simulink model "BO_realisation"  (R2021a)
settings: Solver=FixedStepAuto  StartTime=0.0  StopTime=inf  FixedStep=0.1  RelTol=1e-3  EnableMultiTasking=on
InitFcn:
  | Ts=0.1;
undefined symbols (not defined in the file): sigbuilder_block
libraries: simulink x2, arduinolib x2
settings Model: SimulationMode=external  SILPILModeSetting=veronly  ExtModeTrigDuration=2  Creator=PHAN DU  LastModifiedBy=anass
settings SolverCC: AlgebraicLoopSolver=TrustRegion  AutoInsertRateTranBlk=on
settings DataIOCC: ReturnWorkspaceOutputs=off
settings OptimizationCC: EnhancedBackFolding=on  PassReuseOutputArgsAs=Individual arguments  ZeroExternalMemoryAtStartup=off  ZeroInternalMemoryAtStartup=off  MaxStackSize=64  OptimizeBlockOrder=speed  DifferentSizesBufferReuse=on  EfficientTunableParamExpr=on
settings DebuggingCC: ParameterTunabilityLossMsg=error  SFMachineParentedDataDiag=warning
settings HardwareCC: ProdBitPerInt=16  ProdBitPerPointer=16  ProdBitPerSizeT=16  ProdBitPerPtrDiffT=16  ProdLargestAtomicFloat=None  ProdWordSize=8  ProdHWDeviceType=Atmel->AVR
settings SFSimCC: MATLABDynamicMemAlloc=off
settings RTWCC: SystemTargetFile=ert.tlc  HardwareBoard=Arduino Mega 2560  TemplateMakefile=ert_default_tmf  Toolchain=Arduino AVR  BuildConfiguration=Faster Runs
settings CodeAppCC: ForceParamTrailComments=on  IgnoreCustomStorageClasses=off  OperatorAnnotations=on  SimulinkDataObjDesc=on  SFDataObjDesc=on  InsertBlockDesc=on
settings ERTTargetCC: SupportContinuousTime=on  SupportVariableSizeSignals=on  ExtMode=on  ExtModeStaticAllocSize=2048  ExtModeMexArgs='127.0.0.1' 0 17725

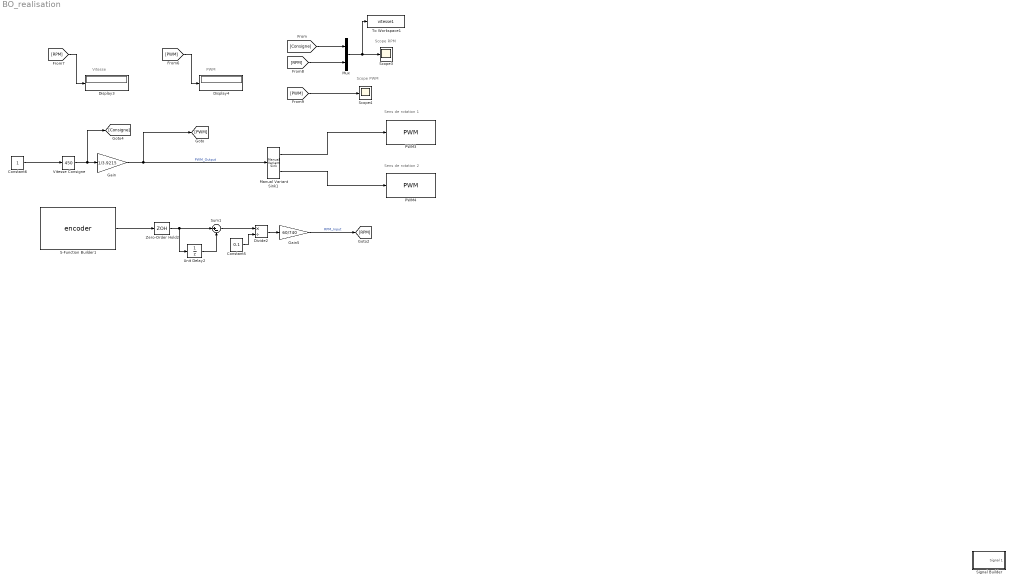
== system BO_realisation ==
  note: Scope PWM
  note: PWM
  note: Vitesse
  note: Scope RPM
  note: Sens de rotation 1
  note: Sens de rotation 2
  Constant5 : Constant  Value=0.1  SampleTime=0.1
  Constant6 : Constant
  Display3 : Display
  Display4 : Display
  Divide2 : Product  Inputs=*/
  Gain : Gain  Gain=1/3.9215
  Gain5 : Gain  Gain=60/740
  Manual Variant Sink1 : simulink/Signal Routing/Manual Variant Sink  NumChoices=2  LabelModeActiveChoice=V_2
  Mux : Mux  Inputs=2
  PWM3 : arduinolib/PWM  pinNumber=5  frequencyType=Default  desiredFrequency=490.2  achievableFrequency=2
  PWM4 : arduinolib/PWM  pinNumber=6  frequencyType=Default  desiredFrequency=490.2  achievableFrequency=2
  S-Function Builder1 : S-Function  InitFcn=try, set_param(gcb,'FunctionName','encoder'), end  FunctionName=encoder  Parameters=int8(0),int8(2),int8(3)  SFunctionModules=encoder_wrapper  SFunctionDeploymentMode=off  EnableBusSupport=off  mask(S-Function Builder){}
      mask help: Simulink:masks:SFunctionBuilder_MD
      mask init:
      | val = [[.9  0.75 0.75 1 1 .9 .9 1]',[1 1 0.75 0.75 .9 .9 1 .9]'];try , sys = get_param(gcb,'SfunBuilderFcnName');if isempty(sys), sys = get_param(gcb,'FunctionName'); end,catch, sys = get_param(gcb,'FunctionName'); end
      settings: CopyFcn=set_param(gcbh,'LinkStatus','none')  PreSaveFcn=try, set_param(gcb,'FunctionName','encoder'), end  OpenFcn=sfunctionwizard(gcbh)
      mask Display:
      | plot(val(:,1),val(:,2))
      | disp(sys)
      | port_label('output',1,'pos')
  Scope3 : Scope
  Scope4 : Scope
  Sum1 : Sum  Inputs=|+-
  To Workspace1 : ToWorkspace  VariableName=vitesse1  SaveFormat=Timeseries  SampleTime=-1
  Unit Delay2 : UnitDelay  SampleTime=-1  HasFrameUpgradeWarning=on
  "Vitesse Consigne " : simulink/Math Operations/Slider Gain  gain=450  low=0  high=1000
  Zero-Order Hold2 : ZeroOrderHold  SampleTime=0.1
  Signal Builder : Subsystem  Tag=STV Subsys  IOType=siggen  LoadFcn=sigbuilder_block('load');  StartFcn=sigbuilder_block('start');  StopFcn=sigbuilder_block('stop');  ClipboardFcn=sigbuilder_block('clipboard');  mask(Sigbuilder block){tuvar=[0:10]}
      mask help: Sigbuilder GUI
      mask init:
      | if ~strcmp(get_param(bdroot(gcbh),'SimulationStatus'),'stopped') tuvar = sigbuilder_block('maskInit'); end
      settings: CopyFcn=sigbuilder_block('copy');  DeleteFcn=sigbuilder_block('delete');  ModelCloseFcn=sigbuilder_block('modelClose');  PreSaveFcn=sigbuilder_block('preSave');  PauseFcn=sigbuilder_block('pause');  ContinueFcn=sigbuilder_block('continue');  NameChangeFcn=sigbuilder_block('namechange');  OpenFcn=sigbuilder_block('open',[437.6 199.2 550.4 400 ]);  CloseFcn=sigbuilder_block('close');
      mask Display: plot(0, 0, 100, 100,[2, 2, 32, 32, 2], [68, 8, 8, 68, 68],[32, 2], [38, 38], [32, 19, 2],[53, 60, 44], [32, 17, 17, 2],[16, 16, 31, 31]);txt = getActiveGroup(gcbh);text(2, 100, txt,'verticalAlignment', 'top');
  wires:
  Sum1/1 -> Divide2/1
  Gain5/1 -> [RPM]  "RPM_Input"
  Unit Delay2/1 -> Sum1/2
  Divide2/1 -> Gain5/1
  S-Function Builder1/1 -> Zero-Order Hold2/1
  [PWM] -> Display4/1
  Constant5/1 -> Divide2/2
  [PWM] -> Scope4/1
  Zero-Order Hold2/1 -> Sum1/1, Unit Delay2/1
  [RPM] -> Display3/1
  Constant6/1 -> "Vitesse Consigne "/1
  [Consigne] -> Mux/1
  [RPM] -> Mux/2
  "Vitesse Consigne "/1 -> [Consigne], Gain/1
  Manual Variant Sink1/2 -> PWM4/1
  Gain/1 -> Manual Variant Sink1/1, [PWM]  "PWM_Output"
  Manual Variant Sink1/1 -> PWM3/1
  Mux/1 -> To Workspace1/1, Scope3/1

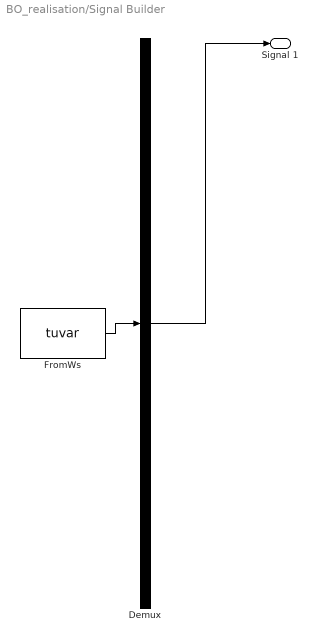
== system BO_realisation/Signal Builder ==
  Demux : Demux  Tag=STV Demux  Outputs=1
      settings: DisplayOption=none
  FromWs : FromWorkspace  Tag=STV FromWs  VariableName=tuvar
      SigBuilderData=|
      | common.afterFinalStr = 'Extrapolate'
      | common.sampleTime = 0
      | dataSet.timeRange = [0 10]
      | dataSet.name = 'Group 1'
      | sbobj.Groups.Name = 'Group 1'
      | sbobj.Groups.Signals.Name = 'Signal 1'
      | sbobj.Groups.Signals.XData = [0 4 4 6 6 10]
      | sbobj.Groups.Signals.YData = [0 0 1 1 0 0]
  Signal 1 : Outport  Tag=STV Outport
  wires:
  FromWs/1 -> Demux/1
  Demux/1 -> Signal 1/1
